simulink model "cubewithpanels0_pd"  (R2022b)
settings: Solver=VariableStepAuto  StartTime=0.0  StopTime=2000  RelTol=1e-3  AbsTol=1e-3
undefined symbols (not defined in the file or in its folder): Angle, Axis
libraries: robotcorelib x2
settings Model: Creator=Abhijit  LastModifiedBy=abhij
settings SolverCC: AutoScaleAbsTol=off  AlgebraicLoopSolver=TrustRegion  MaxZcPerStep=1
settings DebuggingCC: UnconnectedInputMsg=warning  UnconnectedOutputMsg=warning  UnconnectedLineMsg=warning  SymbolicDimsDataTypeCodeGenerationDiagnostic=none  SFMachineParentedDataDiag=warning
settings ModelReferenceCC: EnableRefExpFcnMdlSchedulingChecks=on
settings SFSimCC: CustomCodeUndefinedFunction=UseInterfaceOnly
settings RTWCC: DLArmComputeVersion=19.05
settings SimscapeCC: SimscapeLogType=all  SimscapeLogSimulationStatistics=on  SimscapeLogDataHistory=10000

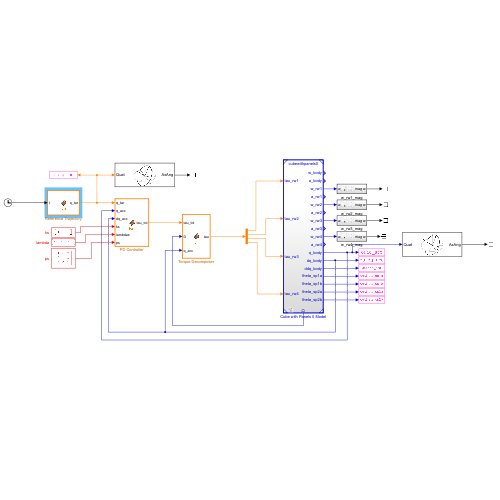
[thumbnail: Simulink's stored preview of the top-level diagram]
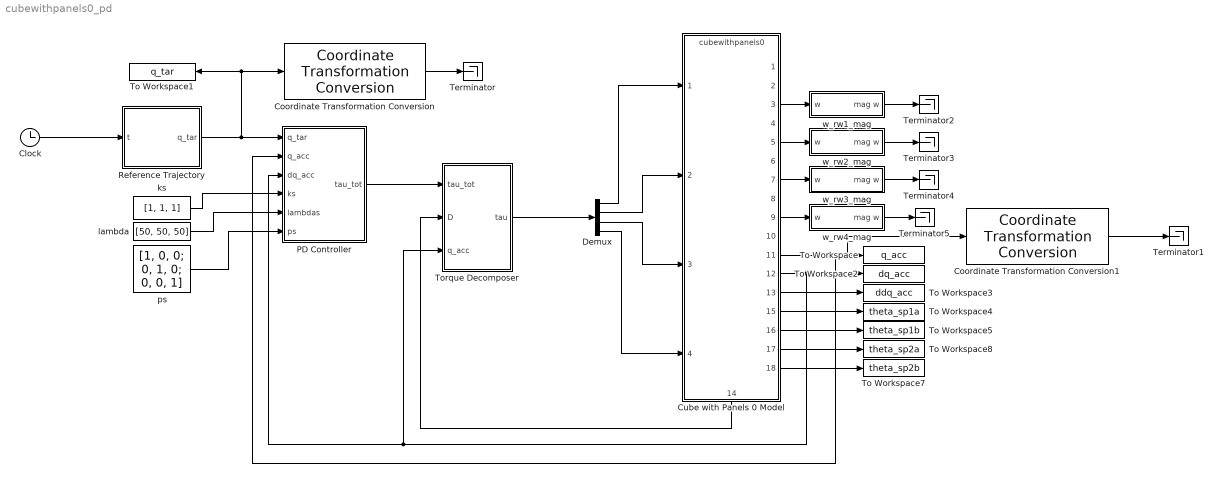
== system cubewithpanels0_pd ==
  Clock : Clock
  Coordinate Transformation Conversion : robotcorelib/Coordinate Transformation Conversion  InputRepresentation=Quaternion  InputEulerSequence=ZYX  ShowTrVecInputPort=on  OutputRepresentation=Axis-Angle  OutputEulerSequence=ZYX  ShowTrVecOutputPort=on  SimulateUsing=Interpreted execution
      settings: LibrarySourceBlock=navlib/Utilities/Coordinate Transformation Conversion
  Coordinate Transformation Conversion1 : robotcorelib/Coordinate Transformation Conversion  InputRepresentation=Quaternion  InputEulerSequence=ZYX  ShowTrVecInputPort=on  OutputRepresentation=Axis-Angle  OutputEulerSequence=ZYX  ShowTrVecOutputPort=on  SimulateUsing=Interpreted execution
      settings: LibrarySourceBlock=navlib/Utilities/Coordinate Transformation Conversion
  Cube with Panels 0 Model : ModelReference  ModelNameDialog=cubewithpanels0.slx  SimulationMode=Normal  ModelReferenceVersion=1.7
      settings: PortSchema="{\"entries\":[{\"content\":{\"sides\":[{\"content\":{\"connectorIds\":[\"In1\",\"In2\",\"In3\",\"In4\"]},\"type\":\"ConnectorPlacement.EquallySpacedRectSide\",\"uuid\":\"8e9d2764-0c8c-4b35-a6b5-330d2d8aade7\"},{\"content\":{\"connectorIds\":[\"Out1\",\"Out2\",\"Out3\",\"Out4\",\"Out5\",\"Out6\",\"Out7\",\"Out8\",\"Out9\",\"Out10\",\"Out11\",\"Out12\",\"Out13\",\"Out15\",\"Out16\",\"Out17\",\"Out18\"],\"side\":\"RIGHT\"},\"type\":\"ConnectorPlacement.EquallySpacedRectSide\",\"uuid\":\"d11583f7-9081-4803-9c4e-bf58094124c2\"},{\"content\":{\"connectorIds\":[],\"side\":\"TOP\"},\"type\":\"ConnectorPlacement.EquallySpacedRectSide\",\"uuid\":\"f987c09c-5813-428e-a812-016ca0940eea\"},{\"content\":{\"connectorIds\":[\"Out14\"],\"side\":\"BOTTOM\"},\"type\":\"ConnectorPlacement.EquallySpacedRectSide\",\"uuid\":\"56fa612c-373e-46c3-86f2-ebb8be87bff3\"}]},\"type\":\"ConnectorPlacement.EquallySpacedConnector\",\"uuid\":\"9c548295-d181-4ae3-baad-4641f0a6e641\"}],\"packageUris\":[\"http://schema.mathworks.com/mf0/Connector/R2020b\"],\"version\":\"1.0\"}"
  Demux : Demux
  PD Controller : MATLAB Function  TreatAsAtomicUnit=on
  Reference Trajectory : MATLAB Function  TreatAsAtomicUnit=on
  Terminator{,1..5} (6 alike) : Terminator
  To Workspace : ToWorkspace  VariableName=q_acc  SaveFormat=Timeseries  SampleTime=-1
  To Workspace1 : ToWorkspace  VariableName=q_tar  SaveFormat=Timeseries  SampleTime=-1
  To Workspace2 : ToWorkspace  VariableName=dq_acc  SaveFormat=Timeseries  SampleTime=-1
  To Workspace3 : ToWorkspace  VariableName=ddq_acc  SaveFormat=Timeseries  SampleTime=-1
  To Workspace4 : ToWorkspace  VariableName=theta_sp1a  SaveFormat=Timeseries  SampleTime=-1
  To Workspace5 : ToWorkspace  VariableName=theta_sp1b  SaveFormat=Timeseries  SampleTime=-1
  To Workspace7 : ToWorkspace  VariableName=theta_sp2b  SaveFormat=Timeseries  SampleTime=-1
  To Workspace8 : ToWorkspace  VariableName=theta_sp2a  SaveFormat=Timeseries  SampleTime=-1
  Torque Decomposer : MATLAB Function  TreatAsAtomicUnit=on
  ks : Constant  Value=[1, 1, 1]
  lambda : Constant  Value=[50, 50, 50]
  ps : Constant  Value=[1, 0, 0; 0, 1, 0; 0, 0, 1]
  w_rw1_mag : Subsystem
  w_rw2_mag : Subsystem
  w_rw3_mag : Subsystem
  w_rw4_mag : Subsystem
  wires:
  Clock/1 -> Reference Trajectory/1(t)
  lambda/1 -> PD Controller/5(lambdas)
  ks/1 -> PD Controller/4(ks)
  ps/1 -> PD Controller/6(ps)
  Reference Trajectory/1(q_tar) -> Coordinate Transformation Conversion/1, To Workspace1/1, PD Controller/1(q_tar)
  Cube with Panels 0 Model/13 -> To Workspace3/1
  Cube with Panels 0 Model/11 -> PD Controller/2(q_acc), Coordinate Transformation Conversion1/1, To Workspace/1
  Cube with Panels 0 Model/15 -> To Workspace4/1
  Cube with Panels 0 Model/16 -> To Workspace5/1
  Cube with Panels 0 Model/17 -> To Workspace8/1
  Cube with Panels 0 Model/18 -> To Workspace7/1
  Torque Decomposer/1(tau) -> Demux/1
  Demux/1 -> Cube with Panels 0 Model/1
  Demux/2 -> Cube with Panels 0 Model/2
  Demux/3 -> Cube with Panels 0 Model/3
  Demux/4 -> Cube with Panels 0 Model/4
  Cube with Panels 0 Model/12 -> To Workspace2/1, Torque Decomposer/3(q_acc), PD Controller/3(dq_acc)
  PD Controller/1(tau_tot) -> Torque Decomposer/1(tau_tot)
  Cube with Panels 0 Model/14 -> Torque Decomposer/2(D)
  w_rw3_mag/1(mag w) -> Terminator4/1
  w_rw4_mag/1(mag w) -> Terminator5/1
  w_rw1_mag/1(mag w) -> Terminator2/1
  Coordinate Transformation Conversion1/1 -> Terminator1/1
  Coordinate Transformation Conversion/1 -> Terminator/1
  w_rw2_mag/1(mag w) -> Terminator3/1
  Cube with Panels 0 Model/3 -> w_rw1_mag/1(w)
  Cube with Panels 0 Model/5 -> w_rw2_mag/1(w)
  Cube with Panels 0 Model/7 -> w_rw3_mag/1(w)
  Cube with Panels 0 Model/9 -> w_rw4_mag/1(w)

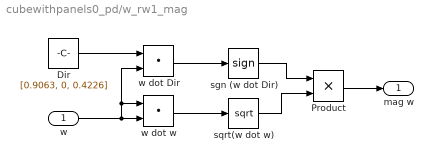
== system cubewithpanels0_pd/w_rw1_mag ==
  w : Inport
  Dir : Constant  Value=[0.9063, 0, 0.4226]
  Product : Product
  sgn (w dot Dir) : Signum
  sqrt(w dot w) : Sqrt
  w dot Dir : DotProduct  OutDataTypeStr=Inherit: Inherit via internal rule
  w dot w : DotProduct  OutDataTypeStr=Inherit: Inherit via internal rule
  mag w : Outport
  wires:
  w dot Dir/1 -> sgn (w dot Dir)/1
  w/1 -> w dot Dir/2, w dot w/1, w dot w/2
  w dot w/1 -> sqrt(w dot w)/1
  Product/1 -> mag w/1
  sqrt(w dot w)/1 -> Product/2
  Dir/1 -> w dot Dir/1
  sgn (w dot Dir)/1 -> Product/1

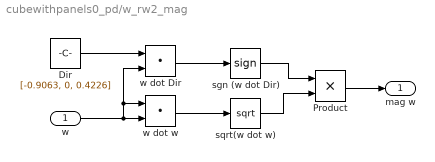
== system cubewithpanels0_pd/w_rw2_mag ==
  w : Inport
  Dir : Constant  Value=[-0.9063, 0, 0.4226]
  Product : Product
  sgn (w dot Dir) : Signum
  sqrt(w dot w) : Sqrt
  w dot Dir : DotProduct  OutDataTypeStr=Inherit: Inherit via internal rule
  w dot w : DotProduct  OutDataTypeStr=Inherit: Inherit via internal rule
  mag w : Outport
  wires:
  w/1 -> w dot Dir/2, w dot w/1, w dot w/2
  w dot w/1 -> sqrt(w dot w)/1
  Product/1 -> mag w/1
  sqrt(w dot w)/1 -> Product/2
  Dir/1 -> w dot Dir/1
  w dot Dir/1 -> sgn (w dot Dir)/1
  sgn (w dot Dir)/1 -> Product/1

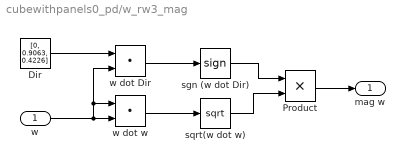
== system cubewithpanels0_pd/w_rw3_mag ==
  w : Inport
  Dir : Constant  Value=[0, 0.9063, 0.4226]
  Product : Product
  sgn (w dot Dir) : Signum
  sqrt(w dot w) : Sqrt
  w dot Dir : DotProduct  OutDataTypeStr=Inherit: Inherit via internal rule
  w dot w : DotProduct  OutDataTypeStr=Inherit: Inherit via internal rule
  mag w : Outport
  wires:
  w/1 -> w dot Dir/2, w dot w/1, w dot w/2
  w dot w/1 -> sqrt(w dot w)/1
  Product/1 -> mag w/1
  sqrt(w dot w)/1 -> Product/2
  Dir/1 -> w dot Dir/1
  w dot Dir/1 -> sgn (w dot Dir)/1
  sgn (w dot Dir)/1 -> Product/1

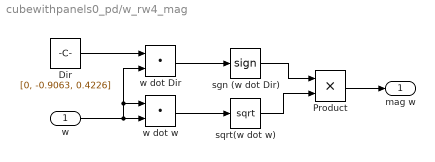
== system cubewithpanels0_pd/w_rw4_mag ==
  w : Inport
  Dir : Constant  Value=[0, -0.9063, 0.4226]
  Product : Product
  sgn (w dot Dir) : Signum
  sqrt(w dot w) : Sqrt
  w dot Dir : DotProduct  OutDataTypeStr=Inherit: Inherit via internal rule
  w dot w : DotProduct  OutDataTypeStr=Inherit: Inherit via internal rule
  mag w : Outport
  wires:
  w/1 -> w dot Dir/2, w dot w/1, w dot w/2
  w dot w/1 -> sqrt(w dot w)/1
  Product/1 -> mag w/1
  sqrt(w dot w)/1 -> Product/2
  Dir/1 -> w dot Dir/1
  w dot Dir/1 -> sgn (w dot Dir)/1
  sgn (w dot Dir)/1 -> Product/1

== matlab function cubewithpanels0_pd/PD Controller ==
  data: tau_tot output; q_tar input; q_acc input; dq_acc input; ks input; lambdas input; ps input
function tau_tot = fcn(q_tar, q_acc, dq_acc, ks, lambdas, ps)
    tau_tot = pdcontroller(q_tar, q_acc, dq_acc, ks, lambdas, ps);

== matlab function cubewithpanels0_pd/Reference Trajectory ==
  settings: updateMethod=CONTINUOUS
  data: t input; q_tar output
function q_tar = fcn(t)
     q_tar = refpath(t, 1);
end

== matlab function cubewithpanels0_pd/Torque Decomposer ==
  data: tau_tot input; tau output; D input; q_acc input
function tau = fcn(tau_tot, D, q_acc)
    tau = taudecomp(tau_tot, D, q_acc);
end
